simulink library "tqd"  (R2021b)
settings: Solver=VariableStepAuto  StartTime=0.0  StopTime=10.0  RelTol=1e-3
undefined symbols (not defined in the file): ATQD_AfterTqMinGain_X_Deg, ATQD_APSCreepBaseTqD_X_kph, ATQD_APSCreepBaseTqD_Y_Deg, ATQD_APSCreepBaseTqR_X_kph, ATQD_APSCreepBaseTqR_Y_Deg, ATQD_APSCreepIterm_X_kph, ATQD_APSCreepIterm_Y_kph, ATQD_APSCreepPterm_X_kph, ATQD_APSCreepPterm_Y_kph, ATQD_APSDecReq_X_kph, ATQD_APSDecReq_Y_mps2, ATQD_APSDecReqCMD_X_kph, ATQD_APSDecReqTs_X_pct, ATQD_APSDecTimeGain_X_Deg, ATQD_APSDecTimeGain_Y_s, ATQD_APSReqLowSpd_X_Deg, ATQD_AutoHoldReleaseBPS_X_Deg, ATQD_AWDLoadTrqnsGain_X_kg, ATQD_AWDLoadTrqnsGain_Y_pct, ATQD_BOSEnBPSPosn_X_kph, ATQD_BOSMap_X_rpm, ATQD_BOSMap_Y_pct, ATQD_CreepBaseTqD_X_kph, ATQD_CreepBaseTqD_Y_Deg, ATQD_CreepBaseTqR_X_kph, ATQD_CreepBaseTqR_Y_Deg, ATQD_CreepBPSDisPosn_X_Deg, ATQD_CreepBPSDisPosnR_X_Deg, ATQD_CreepBPSEnPosn_X_Deg, ATQD_CreepBPSEnPosnR_X_Deg, ATQD_CreepDeltaTq_X_kph, ATQD_CreepIterm_X_kph, ATQD_CreepIterm_Y_kph, ATQD_CreepItermMaxLimit_X_pct, ATQD_CreepPreloadTime_X_kph, ATQD_CreepPreloadTq_X_kph, ATQD_CreepPreloadTq_Y_s, ATQD_CreepProtTq_X_Deg, ATQD_CreepPterm_X_kph, ATQD_CreepPterm_Y_kph, ATQD_CreepRrTqSpRat_X_rpm, ATQD_CreepRrTqSpRat_Y_Nm, ATQD_CreepTargetSpdD_X_pct, ATQD_CreepTargetSpdR_X_pct, ATQD_ECOTqMapD_X_rpm, ATQD_ECOTqMapD_Y_pct, ATQD_EMTqMapD_X_rpm, ATQD_EMTqMapD_Y_pct, ATQD_EOPDTqMapDCon_X_rpm, ATQD_EOPDTqMapDCon_Y_Deg, ATQD_EscapeModePedTq_X_pct, ATQD_EscapeModePedTq_Y_rpm, ATQD_EscapeModePedTqFr_X_pct, ATQD_EscapeModePedTqFr_Y_rpm, ATQD_EstInitVehWeight_X_c, ATQD_FAfterTqCMDGain_X_rpm, ATQD_FAfterTqCMDGain_Y_pct, ATQD_FrLossMAPLowV_X_rpm, ATQD_FrLossMAPLowV_Y_Nm, ATQD_FrMotActReduce_X_rpm ... (+772)
libraries: simulink x211, hcu_lib x179, tqr x3
(part 19 of 28)

== system tqd/TQD/TorqueDemand/TorqueModule/AvaliableTqLimit/TorqueCapacityCalcalation/Generation ==
  VTQD_FrShaftSpd_rpm : Inport
  VTQD_RrShaftSpd_rpm : Inport  Port=2
  VTQD_FrHVBPwrAvailChrg_kw : Inport  Port=3
  VTQD_RrHVBPwrAvailChrg_kw : Inport  Port=4
  KTQD_FrBatapCont_factor : Inport  Port=5
  KTQD_RrBatapCont_factor : Inport  Port=6
  VINP_FrRegenAvailTq_Nm : Inport  Port=7
  VINP_RrRegenAvailTq_Nm : Inport  Port=8
  VTQD_GearActualPosn_enum : Inport  Port=9
  VINP_VehicleType_enum : Inport  Port=10
  VTQD_FrMotorTempHigh_flg : Inport  Port=11
  VTQD_RrMotorTempHigh_flg : Inport  Port=12
  VTQD_FrGenActReduce_Nm : Inport  Port=13
  VTQD_RrGenActReduce_Nm : Inport  Port=14
  Abs2 : Abs
  Abs6 : Abs
  Constant : Constant  Value=KTQD_WhlTqCapGenFr_Nm_ovrdflg
  Constant1 : Constant  Value=KTQD_WhlTqCapGenFr_Nm_ovrdval
  Constant10 : Constant  Value=ENUM_GEARACTUALPOSN_P  OutDataTypeStr=single
  Constant11 : Constant  Value=ENUM_VEHICLETYPE_D31L24
  Constant12 : Constant  Value=KTQD_RrLowTheldTrq_Nm  OutDataTypeStr=single
  Constant13 : Constant  Value=ZERO_FLOAT
  Constant14 : Constant  Value=KTQD_FrLowTheldTrq_Nm  OutDataTypeStr=single
  Constant15 : Constant  Value=KTQD_NewTotalCapTqSW_flg
  Constant16 : Constant  Value=ENUM_GEARACTUALPOSN_N  OutDataTypeStr=single
  Constant17 : Constant  Value=ENUM_GEARACTUALPOSN_P  OutDataTypeStr=single
  Constant18 : Constant  Value=KTQD_FrLowTheldTrq_Nm
  Constant19 : Constant  Value=ENUM_VEHICLETYPE_D31L24
  Constant2 : Constant  Value=KTQD_RrTMSpdMin_rpm  OutDataTypeStr=single
  Constant24 : Constant  Value=KTQD_NewTotalCapTqSW_flg
  Constant25 : Constant  Value=KTQD_RrLowTheldTrq_Nm
  Constant3 : Constant  Value=KTQD_WhlTqCapGenRr_Nm_ovrdflg
  Constant4 : Constant  Value=KTQD_RrTMTotalGearRatio_gain  OutDataTypeStr=single
  Constant5 : Constant  Value=KTQD_FrTMSpdMin_rpm  OutDataTypeStr=single
  Constant6 : Constant  Value=KTQD_FrTMTotalGearRatio_gain  OutDataTypeStr=single
  Constant7 : Constant  Value=KTQD_WhlTqCapGenRr_Nm_ovrdval
  Constant8 : Constant  Value=ZERO_FLOAT
  Constant9 : Constant  Value=ENUM_GEARACTUALPOSN_N  OutDataTypeStr=single
  Equal{1..4} (4 alike) : RelationalOperator  Operator===  OutDataTypeStr=boolean  RndMeth=Simplest
  Equal5 : RelationalOperator  Operator=~=  OutDataTypeStr=boolean  RndMeth=Simplest
  Equal6 : RelationalOperator  Operator=~=  OutDataTypeStr=boolean  RndMeth=Simplest
  Fcn : Fcn  Expr=u[1]/u[2]/pi*u[3]
  Fcn2 : Fcn  Expr=u[1]/u[2]/pi*u[3]
  Gain1 : Gain  Gain=-1
  Gain4 : Gain  Gain=-1
  Logical Operator1 : Logic  AllPortsSameDT=off  OutDataTypeStr=boolean
  Logical Operator2 : Logic  AllPortsSameDT=off  OutDataTypeStr=boolean
  Max{,1..5} (6 alike) : MinMax  Function=max  Inputs=2
  Mux : Mux  Inputs=3
  Mux2 : Mux  Inputs=3
  OR1 : Logic  Operator=OR  AllPortsSameDT=off  OutDataTypeStr=boolean
  OR2 : Logic  Operator=OR  AllPortsSameDT=off  OutDataTypeStr=boolean
  Product1 : Product
  Product2 : Product
  Saturation1 : Saturate  UpperLimit=0  LowerLimit=KTQD_FrLowTheldTrq_Nm
      settings: AttributesFormatString=|
      | Upper Limit :%<UpperLimit>
      | Lower Limit :%<LowerLimit>
  Saturation2 : Saturate  UpperLimit=0  LowerLimit=KTQD_RrLowTheldTrq_Nm
      settings: AttributesFormatString=|
      | Upper Limit :%<UpperLimit>
      | Lower Limit :%<LowerLimit>
  Switch{,1,6..7} (4 alike) : Switch  Criteria=u2 ~= 0
      Switch settings: AttributesFormatString=<%<Criteria>>
      Switch1 settings: AttributesFormatString=<%<Criteria>>
      Switch6 settings: AttributesFormatString=%<Criteria>
      Switch7 settings: AttributesFormatString=%<Criteria>
  Switch{2..5} (4 alike) : Switch  Criteria=u2 > Threshold
  VTQD_WhlTqCapGenFr_Nm : Outport
  VTQD_WhlTqCapGenRr_Nm : Outport  Port=2
  wires:
  Gain1/1 -> Saturation2/1
  Gain4/1 -> Saturation1/1
  Switch1/1 -> VTQD_WhlTqCapGenRr_Nm/1  "VTQD_WhlTqCapGenRr_Nm"
  Constant3/1 -> Switch1/2
  Constant7/1 -> Switch1/1
  Switch/1 -> VTQD_WhlTqCapGenFr_Nm/1  "VTQD_WhlTqCapGenFr_Nm"
  Constant1/1 -> Switch/1
  Constant/1 -> Switch/2
  VTQD_RrHVBPwrAvailChrg_kw/1 -> [VTQD_RrHVBPwrAvailChrg_kw]
  KTQD_FrBatapCont_factor/1 -> [KTQD_FrBatapCont_factor]
  VTQD_FrHVBPwrAvailChrg_kw/1 -> [VTQD_FrHVBPwrAvailChrg_kw]
  VTQD_FrShaftSpd_rpm/1 -> [VTQD_FrShaftSpd_rpm]
  VTQD_RrShaftSpd_rpm/1 -> [VTQD_RrShaftSpd_rpm]
  KTQD_RrBatapCont_factor/1 -> [KTQD_RrBatapCont_factor]
  Fcn2/1 -> Gain1/1
  Max1/1 -> Mux2/2
  Abs2/1 -> Max1/1
  Mux2/1 -> Fcn2/1
  Constant2/1 -> Max1/2
  [KTQD_RrBatapCont_factor] -> Mux2/3
  [VTQD_RrShaftSpd_rpm] -> Abs2/1
  [VTQD_RrHVBPwrAvailChrg_kw] -> Mux2/1
  Abs6/1 -> Max4/1
  [VTQD_FrHVBPwrAvailChrg_kw] -> Mux/1
  Constant5/1 -> Max4/2
  [VTQD_FrShaftSpd_rpm] -> Abs6/1
  [KTQD_FrBatapCont_factor] -> Mux/3
  Mux/1 -> Fcn/1
  Max4/1 -> Mux/2
  [VINP_FrRegenAvailTq_Nm] -> Product2/1
  Constant6/1 -> Product2/2
  [VINP_RrRegenAvailTq_Nm] -> Product1/1
  Constant4/1 -> Product1/2
  VINP_RrRegenAvailTq_Nm/1 -> [VINP_RrRegenAvailTq_Nm]
  VINP_FrRegenAvailTq_Nm/1 -> [VINP_FrRegenAvailTq_Nm]
  [VTQD_GearActualPosn_enum] -> Equal3/1
  Equal3/1 -> OR1/1
  Constant17/1 -> Equal3/2
  [VTQD_GearActualPosn_enum] -> Equal1/1
  Constant13/1 -> Switch3/1
  Equal1/1 -> OR1/2
  Constant16/1 -> Equal1/2
  Switch3/1 -> Max/2
  Constant8/1 -> Switch2/1
  [VTQD_GearActualPosn_enum] -> Equal2/1
  Constant10/1 -> Equal4/2
  Equal4/1 -> OR2/1
  Constant9/1 -> Equal2/2
  Equal2/1 -> OR2/2
  [VTQD_GearActualPosn_enum] -> Equal4/1
  Switch2/1 -> Max2/2
  VTQD_GearActualPosn_enum/1 -> [VTQD_GearActualPosn_enum]
  Max/1 -> Switch1/3
  Max2/1 -> Switch/3
  VINP_VehicleType_enum/1 -> [VINP_VehicleType_enum]
  Equal6/1 -> Logical Operator1/2
  [VINP_VehicleType_enum] -> Equal6/1
  Constant19/1 -> Equal6/2
  Logical Operator1/1 -> Switch2/2
  OR2/1 -> Logical Operator1/1
  [VINP_VehicleType_enum] -> Equal5/1
  Constant11/1 -> Equal5/2
  Equal5/1 -> Logical Operator2/2
  Logical Operator2/1 -> Switch3/2
  OR1/1 -> Logical Operator2/1
  VTQD_FrMotorTempHigh_flg/1 -> [VTQD_FrMotorTempHigh_flg]
  VTQD_RrMotorTempHigh_flg/1 -> [VTQD_RrMotorTempHigh_flg]
  VTQD_FrGenActReduce_Nm/1 -> [VTQD_FrGenActReduce_Nm]
  VTQD_RrGenActReduce_Nm/1 -> [VTQD_RrGenActReduce_Nm]
  [VTQD_RrGenActReduce_Nm] -> Switch4/1
  [VTQD_RrMotorTempHigh_flg] -> Switch4/2
  Product1/1 -> Max5/1
  Switch4/1 -> Max5/2
  Max5/1 -> Switch3/3
  [VTQD_FrMotorTempHigh_flg] -> Switch5/2
  [VTQD_FrGenActReduce_Nm] -> Switch5/1
  Max3/1 -> Switch2/3
  Product2/1 -> Max3/1
  Switch5/1 -> Max3/2
  Fcn/1 -> Gain4/1
  Constant14/1 -> Switch5/3
  Constant12/1 -> Switch4/3
  Constant25/1 -> Switch7/1
  Constant24/1 -> Switch7/2
  Saturation2/1 -> Switch7/3
  Switch7/1 -> Max/1
  Constant18/1 -> Switch6/1
  Constant15/1 -> Switch6/2
  Saturation1/1 -> Switch6/3
  Switch6/1 -> Max2/1

== system tqd/TQD/TorqueDemand/TorqueModule/AvaliableTqLimit/TorqueCapacityCalcalation/MOTOR Loss MAP  ==
  note: Determination
  note: Front Loss Power Calculation
  note: Calabration Parameters/Maps
  note: Rear Loss Power Calculation
  VTQD_FrShaftSpd_rpm : Inport
  VTQD_RrShaftSpd_rpm : Inport  Port=2
  VTQD_CoordWhlTqDemFr_Nm : Inport  Port=3
  VTQD_CoordWhlTqDemRr_Nm : Inport  Port=4
  VINP_FrMCUDCBusVolt_V : Inport  Port=5
  VINP_RrMCUDCBusVolt_V : Inport  Port=6
  VPMM_DrivetrainSelect_enum : Inport  Port=7
  AND : Logic  AllPortsSameDT=off  OutDataTypeStr=boolean
  AND2 : Logic  AllPortsSameDT=off  OutDataTypeStr=boolean
  Add : Sum
  Add2 : Sum
  Add3 : Sum
  Constant : Constant  Value=KTQD_FrLossMAPLowV_V
  Constant1 : Constant  Value=KTQD_FrLossMAPHighV_V
  Constant10 : Constant  Value=eps  OutDataTypeStr=single
  Constant{6,11..13} (4 alike) : Constant  Value=ZERO_FLOAT
  Constant2 : Constant  Value=KTQD_RrLossMAPLowV_V
  Constant3 : Constant  Value=KTQD_RrLossMAPHighV_V
  Constant4 : Constant  Value=ENUM_DRIVETRAIN_AWD
  Constant5 : Constant  Value=ENUM_DRIVETRAIN_RWD
  Constant7 : Constant  Value=eps  OutDataTypeStr=single
  Divide : Product  Inputs=*/
  Divide2 : Product  Inputs=*/
  Equal : RelationalOperator  Operator===  OutDataTypeStr=boolean  RndMeth=Simplest
  Equal1 : RelationalOperator  Operator===  OutDataTypeStr=boolean  RndMeth=Simplest
  GreaterThan : RelationalOperator  Operator=>  OutDataTypeStr=boolean  RndMeth=Simplest
  GreaterThan2 : RelationalOperator  Operator=>  OutDataTypeStr=boolean  RndMeth=Simplest
  Less Than : RelationalOperator  Operator=<  OutDataTypeStr=boolean  RndMeth=Simplest
  Less Than2 : RelationalOperator  Operator=<  OutDataTypeStr=boolean  RndMeth=Simplest
  MTQD_FrLossMAPHighV_Z_kw : Lookup_n-D  BreakpointsForDimension1=ATQD_FrLossMAPLowV_Y_Nm  BreakpointsForDimension2=ATQD_FrLossMAPLowV_X_rpm  Table=MTQD_FrLossMAPHighV_Z_kw  InternalRulePriority=Speed  RndMeth=Simplest  InputSameDT=on
      settings: InputPortMap=u0,u1
  MTQD_FrLossMAPLowV_Z_kw : Lookup_n-D  BreakpointsForDimension1=ATQD_FrLossMAPLowV_Y_Nm  BreakpointsForDimension2=ATQD_FrLossMAPLowV_X_rpm  Table=MTQD_FrLossMAPLowV_Z_kw  InternalRulePriority=Speed  RndMeth=Simplest  InputSameDT=on
      settings: InputPortMap=u0,u1
  MTQD_RrLossMAPHighV_Z_kw : Lookup_n-D  BreakpointsForDimension1=ATQD_RrLossMAPLowV_Y_Nm  BreakpointsForDimension2=ATQD_RrLossMAPLowV_X_rpm  Table=MTQD_RrLossMAPHighV_Z_kw  InternalRulePriority=Speed  RndMeth=Simplest  InputSameDT=on
      settings: InputPortMap=u0,u1
  MTQD_RrLossMAPLowV_Z_kw : Lookup_n-D  BreakpointsForDimension1=ATQD_RrLossMAPLowV_Y_Nm  BreakpointsForDimension2=ATQD_RrLossMAPLowV_X_rpm  Table=MTQD_RrLossMAPLowV_Z_kw  InternalRulePriority=Speed  RndMeth=Simplest  InputSameDT=on
      settings: InputPortMap=u0,u1
  Max : MinMax  Function=max  Inputs=2
  Max1 : MinMax  Function=max  Inputs=2
  Product : Product
  Product2 : Product
  Subtract{,1..2,6..8} (6 alike) : Sum  Inputs=+-
  Switch : Switch  Criteria=u2 > Threshold
  Switch1 : Switch  Criteria=u2 > Threshold
  Switch3 : Switch  Criteria=u2 ~= 0
  Switch4 : Switch  Criteria=u2 ~= 0
  VTQD_MotorLossTotal_kw : Outport
  wires:
  MTQD_FrLossMAPLowV_Z_kw/1 -> [VTQD_FrLossMAPLowV_kw]  "VTQD_FrLossMAPLowV_kw"
  MTQD_FrLossMAPHighV_Z_kw/1 -> [VTQD_FrLossMAPHighV_kw]  "VTQD_FrLossMAPHighV_kw"
  Constant/1 -> [VTQD_FrLossMAPLowV_V]  "VTQD_FrLossMAPLowV_V"
  Constant1/1 -> [VTQD_FrLossMAPHighV_V]  "VTQD_FrLossMAPHighV_V"
  Constant2/1 -> [VTQD_RrLossMAPLowV_V]  "VTQD_RrLossMAPLowV_V"
  Constant3/1 -> [VTQD_RrLossMAPHighV_V]  "VTQD_RrLossMAPHighV_V"
  MTQD_RrLossMAPLowV_Z_kw/1 -> [VTQD_RrLossMAPLowV_kw]  "VTQD_RrLossMAPLowV_kw"
  MTQD_RrLossMAPHighV_Z_kw/1 -> [VTQD_RrLossMAPHighV_kw]  "VTQD_RrLossMAPHighV_kw"
  VINP_FrMCUDCBusVolt_V/1 -> [VINP_FrMCUDCBusVolt_V]
  VINP_RrMCUDCBusVolt_V/1 -> [VINP_RrMCUDCBusVolt_V]
  [VINP_FrMCUDCBusVolt_V] -> Subtract/1
  [VTQD_FrLossMAPLowV_V] -> Subtract/2
  Subtract/1 -> Divide/1
  Divide/1 -> Product/1
  Product/1 -> Add/1
  [VTQD_FrLossMAPLowV_kw] -> Add/2
  Switch3/1 -> [VTQD_FrLossMAPFinal_kw]  "VTQD_FrLossMAPFinal_kw"
  [VPMM_DrivetrainSelect_enum] -> Equal/1
  Constant4/1 -> Equal/2
  Equal/1 -> Switch/2
  Add2/1 -> Switch/1
  [VPMM_DrivetrainSelect_enum] -> Equal1/1
  Constant5/1 -> Equal1/2
  [VTQD_RrLossMAPFinal_kw] -> Switch1/1
  Switch1/1 -> Switch/3
  [VTQD_FrLossMAPFinal_kw] -> Switch1/3
  Equal1/1 -> Switch1/2
  Switch/1 -> [VTQD_MotorLossTotal_kw]  "VTQD_MotorLossTotal_kw"
  VTQD_CoordWhlTqDemFr_Nm/1 -> [VTQD_CoordWhlTqDemFr_Nm]
  Add/1 -> Switch3/1
  [VTQD_CoordWhlTqDemFr_Nm] -> GreaterThan/1
  Constant6/1 -> GreaterThan/2
  GreaterThan/1 -> AND/1
  Constant11/1 -> Switch3/3
  Less Than/1 -> AND/2
  AND/1 -> Switch3/2
  VTQD_FrShaftSpd_rpm/1 -> [VTQD_FrShaftSpd_rpm]
  VTQD_RrShaftSpd_rpm/1 -> [VTQD_RrShaftSpd_rpm]
  VTQD_CoordWhlTqDemRr_Nm/1 -> [VTQD_CoordWhlTqDemRr_Nm]
  VPMM_DrivetrainSelect_enum/1 -> [VPMM_DrivetrainSelect_enum]
  [VTQD_CoordWhlTqDemFr_Nm] -> MTQD_FrLossMAPLowV_Z_kw/1
  [VTQD_FrShaftSpd_rpm] -> MTQD_FrLossMAPLowV_Z_kw/2
  [VTQD_CoordWhlTqDemFr_Nm] -> MTQD_FrLossMAPHighV_Z_kw/1
  [VTQD_FrShaftSpd_rpm] -> MTQD_FrLossMAPHighV_Z_kw/2
  [VTQD_CoordWhlTqDemRr_Nm] -> MTQD_RrLossMAPLowV_Z_kw/1
  [VTQD_RrShaftSpd_rpm] -> MTQD_RrLossMAPLowV_Z_kw/2
  [VTQD_CoordWhlTqDemRr_Nm] -> MTQD_RrLossMAPHighV_Z_kw/1
  [VTQD_RrShaftSpd_rpm] -> MTQD_RrLossMAPHighV_Z_kw/2
  [VTQD_FrLossMAPLowV_V] -> Subtract1/2
  [VTQD_FrLossMAPHighV_V] -> Subtract1/1
  Subtract1/1 -> Max/1
  Constant10/1 -> Max/2
  Max/1 -> Divide/2
  [VTQD_FrLossMAPLowV_kw] -> Subtract2/2
  [VTQD_FrLossMAPHighV_kw] -> Subtract2/1
  Subtract2/1 -> Product/2
  [VINP_FrMCUDCBusVolt_V] -> Less Than/1
  [VTQD_FrLossMAPHighV_V] -> Less Than/2
  [VTQD_RrLossMAPHighV_V] -> Less Than2/2
  [VINP_RrMCUDCBusVolt_V] -> Less Than2/1
  Subtract8/1 -> Product2/2
  [VTQD_RrLossMAPHighV_kw] -> Subtract8/1
  [VTQD_RrLossMAPLowV_kw] -> Subtract8/2
  Max1/1 -> Divide2/2
  Constant7/1 -> Max1/2
  Subtract7/1 -> Max1/1
  [VTQD_RrLossMAPHighV_V] -> Subtract7/1
  [VTQD_RrLossMAPLowV_V] -> Subtract7/2
  AND2/1 -> Switch4/2
  Less Than2/1 -> AND2/2
  Constant12/1 -> Switch4/3
  GreaterThan2/1 -> AND2/1
  Constant13/1 -> GreaterThan2/2
  [VTQD_CoordWhlTqDemRr_Nm] -> GreaterThan2/1
  Add3/1 -> Switch4/1
  Switch4/1 -> [VTQD_RrLossMAPFinal_kw]  "VTQD_RrLossMAPFinal_kw"
  [VTQD_RrLossMAPLowV_kw] -> Add3/2
  Product2/1 -> Add3/1
  Divide2/1 -> Product2/1
  Subtract6/1 -> Divide2/1
  [VTQD_RrLossMAPLowV_V] -> Subtract6/2
  [VINP_RrMCUDCBusVolt_V] -> Subtract6/1
  [VTQD_FrLossMAPFinal_kw] -> Add2/1
  [VTQD_RrLossMAPFinal_kw] -> Add2/2
  [VTQD_MotorLossTotal_kw] -> VTQD_MotorLossTotal_kw/1

== system tqd/TQD/TorqueDemand/TorqueModule/AvaliableTqLimit/TorqueCapacityCalcalation/Motoring ==
  VTQD_FrShaftSpd_rpm : Inport
  VTQD_RrShaftSpd_rpm : Inport  Port=2
  VTQD_FrHVBPwrAvailDchrg_kw : Inport  Port=3
  VTQD_RrHVBPwrAvailDchrg_kw : Inport  Port=4
  KTQD_FrBatapCont_factor : Inport  Port=5
  KTQD_RrBatapCont_factor : Inport  Port=6
  VINP_FrMotorAvailTq_Nm : Inport  Port=7
  VINP_RrMotorAvailTq_Nm : Inport  Port=8
  VTQD_GearActualPosn_enum : Inport  Port=9
  VINP_VehicleType_enum : Inport  Port=10
  VTQD_FrMotorTempHigh_flg : Inport  Port=11
  VTQD_RrMotorTempHigh_flg : Inport  Port=12
  VTQD_FrMotActReduce_gain : Inport  Port=13
  VTQD_RrMotActReduce_Nm : Inport  Port=14
  VTQD_FrRockDisAvalMotTq_Nm : Inport  Port=15
  VTQD_RrRockDisAvalMotTq_Nm : Inport  Port=16
  Abs : Abs
  Abs2 : Abs
  Constant : Constant  Value=KTQD_WhlTqCapMotFr_Nm_ovrdflg
  Constant1 : Constant  Value=KTQD_FrTMSpdMin_rpm  OutDataTypeStr=single
  Constant10 : Constant  Value=KTQD_FrTMTotalGearRatio_gain  OutDataTypeStr=single
  Constant11 : Constant  Value=KTQD_RrTMTotalGearRatio_gain  OutDataTypeStr=single
  Constant{2,4,12..13} (4 alike) : Constant  Value=ZERO_FLOAT
  Constant14 : Constant  Value=ENUM_GEARACTUALPOSN_N  OutDataTypeStr=single
  Constant15 : Constant  Value=ENUM_GEARACTUALPOSN_P  OutDataTypeStr=single
  Constant16 : Constant  Value=ENUM_GEARACTUALPOSN_N  OutDataTypeStr=single
  Constant17 : Constant  Value=ENUM_GEARACTUALPOSN_P  OutDataTypeStr=single
  Constant18 : Constant  Value=ENUM_VEHICLETYPE_D31L24
  Constant19 : Constant  Value=ENUM_VEHICLETYPE_D31L24
  Constant20 : Constant  Value=KTQD_RrUppTheldTrq_Nm
  Constant21 : Constant  Value=KTQD_FrUppTheldTrq_Nm
  Constant22 : Constant  Value=KTQD_NewTotalCapTqSW_flg
  Constant23 : Constant  Value=KTQD_FrUppTheldTrq_Nm
  Constant24 : Constant  Value=KTQD_NewTotalCapTqSW_flg
  Constant25 : Constant  Value=KTQD_RrUppTheldTrq_Nm
  Constant3 : Constant  Value=KTQD_RrTMSpdMin_rpm  OutDataTypeStr=single
  Constant5 : Constant  Value=KTQD_WhlTqCapMotFr_Nm_ovrdval
  Constant6 : Constant  Value=KTQD_WhlTqCapMotRr_Nm_ovrdflg
  Constant7 : Constant  Value=KTQD_WhlTqCapMotRr_Nm_ovrdval
  Constant8 : Constant  Value=KTQD_FrUppTheldTrq_Nm
  Constant9 : Constant  Value=KTQD_RrUppTheldTrq_Nm
  Equal{,1..3} (4 alike) : RelationalOperator  Operator===  OutDataTypeStr=boolean  RndMeth=Simplest
  Equal4 : RelationalOperator  Operator=~=  OutDataTypeStr=boolean  RndMeth=Simplest
  Equal6 : RelationalOperator  Operator=~=  OutDataTypeStr=boolean  RndMeth=Simplest
  Fcn : Fcn  Expr=u[1]/u[2]/pi*u[3]
  Fcn2 : Fcn  Expr=u[1]/u[2]/pi*u[3]
  Logical Operator1 : Logic  AllPortsSameDT=off  OutDataTypeStr=boolean
  Logical Operator2 : Logic  AllPortsSameDT=off  OutDataTypeStr=boolean
  Max{,1..3} (4 alike) : MinMax  Function=max  Inputs=2
  Min : MinMax  Inputs=4
  Min1 : MinMax  Inputs=4
  Min2 : MinMax  Inputs=2
  Min3 : MinMax  Inputs=2
  Mux : Mux  Inputs=3
  Mux2 : Mux  Inputs=3
  OR : Logic  Operator=OR  AllPortsSameDT=off  OutDataTypeStr=boolean
  OR1 : Logic  Operator=OR  AllPortsSameDT=off  OutDataTypeStr=boolean
  Product : Product
  Product1 : Product
  Switch{,1,6..7} (4 alike) : Switch  Criteria=u2 ~= 0
      Switch settings: AttributesFormatString=<%<Criteria>>
      Switch1 settings: AttributesFormatString=<%<Criteria>>
      Switch6 settings: AttributesFormatString=%<Criteria>
      Switch7 settings: AttributesFormatString=%<Criteria>
  Switch{2..5} (4 alike) : Switch  Criteria=u2 > Threshold
  VTQD_WhlTqCapMotFr_Nm : Outport
  VTQD_WhlTqCapMotRr_Nm : Outport  Port=2
  wires:
  Switch1/1 -> VTQD_WhlTqCapMotRr_Nm/1  "VTQD_WhlTqCapMotRr_Nm"
  Constant7/1 -> Switch1/1
  Constant6/1 -> Switch1/2
  Constant5/1 -> Switch/1
  Constant/1 -> Switch/2
  Switch/1 -> VTQD_WhlTqCapMotFr_Nm/1  "VTQD_WhlTqCapMotFr_Nm"
  VTQD_RrHVBPwrAvailDchrg_kw/1 -> [VTQD_RrHVBPwrAvailDchrg_kw]
  KTQD_RrBatapCont_factor/1 -> [KTQD_RrBatapCont_factor]
  VTQD_RrShaftSpd_rpm/1 -> [VTQD_RrShaftSpd_rpm]
  Abs2/1 -> Max2/1
  [VTQD_RrHVBPwrAvailDchrg_kw] -> Mux2/1
  Constant3/1 -> Max2/2
  [VTQD_RrShaftSpd_rpm] -> Abs2/1
  Mux2/1 -> Fcn2/1
  Max2/1 -> Mux2/2
  [VTQD_FrHVBPwrAvailDchrg_kw] -> Mux/1
  Max/1 -> Mux/2
  [VTQD_FrShaftSpd_rpm] -> Abs/1
  KTQD_FrBatapCont_factor/1 -> [KTQD_FrBatapCont_factor]
  VTQD_FrHVBPwrAvailDchrg_kw/1 -> [VTQD_FrHVBPwrAvailDchrg_kw]
  Abs/1 -> Max/1
  Mux/1 -> Fcn/1
  VTQD_FrShaftSpd_rpm/1 -> [VTQD_FrShaftSpd_rpm]
  Constant1/1 -> Max/2
  Constant8/1 -> Min/2
  Min/1 -> Max1/1
  Constant2/1 -> Max1/2
  Constant9/1 -> Min1/2
  Constant4/1 -> Max3/2
  [KTQD_FrBatapCont_factor] -> Mux/3
  [KTQD_RrBatapCont_factor] -> Mux2/3
  VINP_FrMotorAvailTq_Nm/1 -> [VINP_FrMotorAvailTq_Nm]
  VINP_RrMotorAvailTq_Nm/1 -> [VINP_RrMotorAvailTq_Nm]
  Constant10/1 -> Product/2
  [VINP_FrMotorAvailTq_Nm] -> Product/1
  [VINP_RrMotorAvailTq_Nm] -> Product1/1
  Constant11/1 -> Product1/2
  Min1/1 -> Max3/1
  Constant12/1 -> Switch2/1
  Constant14/1 -> Equal/2
  [VTQD_GearActualPosn_enum] -> Equal/1
  Equal2/1 -> OR/1
  [VTQD_GearActualPosn_enum] -> Equal2/1
  Equal/1 -> OR/2
  Constant15/1 -> Equal2/2
  Equal1/1 -> OR1/2
  Equal3/1 -> OR1/1
  Constant17/1 -> Equal3/2
  [VTQD_GearActualPosn_enum] -> Equal1/1
  Constant16/1 -> Equal1/2
  Constant13/1 -> Switch3/1
  [VTQD_GearActualPosn_enum] -> Equal3/1
  VTQD_GearActualPosn_enum/1 -> [VTQD_GearActualPosn_enum]
  Max1/1 -> Switch/3
  Max3/1 -> Switch1/3
  Constant19/1 -> Equal6/2
  [VINP_VehicleType_enum] -> Equal6/1
  Equal6/1 -> Logical Operator1/2
  VINP_VehicleType_enum/1 -> [VINP_VehicleType_enum]
  Logical Operator1/1 -> Switch2/2
  OR/1 -> Logical Operator1/1
  Equal4/1 -> Logical Operator2/2
  [VINP_VehicleType_enum] -> Equal4/1
  Constant18/1 -> Equal4/2
  Logical Operator2/1 -> Switch3/2
  OR1/1 -> Logical Operator2/1
  VTQD_RrMotActReduce_Nm/1 -> [VTQD_RrMotActReduce_Nm]
  VTQD_FrMotActReduce_gain/1 -> [VTQD_FrMotActReduce_Nm]
  VTQD_RrMotorTempHigh_flg/1 -> [VTQD_RrMotorTempHigh_flg]
  VTQD_FrMotorTempHigh_flg/1 -> [VTQD_FrMotorTempHigh_flg]
  [VTQD_RrMotorTempHigh_flg] -> Switch4/2
  [VTQD_RrMotActReduce_Nm] -> Switch4/1
  Product1/1 -> Min3/1
  Switch4/1 -> Min3/2
  Min3/1 -> Switch3/3
  [VTQD_FrMotorTempHigh_flg] -> Switch5/2
  [VTQD_FrMotActReduce_Nm] -> Switch5/1
  Product/1 -> Min2/1
  Switch5/1 -> Min2/2
  Min2/1 -> Switch2/3
  Constant21/1 -> Switch5/3
  Constant20/1 -> Switch4/3
  VTQD_FrRockDisAvalMotTq_Nm/1 -> [VTQD_FrRockDisAvalMotTq_Nm]
  VTQD_RrRockDisAvalMotTq_Nm/1 -> [VTQD_RrRockDisAvalMotTq_Nm]
  Switch2/1 -> Min/4
  [VTQD_FrRockDisAvalMotTq_Nm] -> Min/3
  Switch3/1 -> Min1/4
  [VTQD_RrRockDisAvalMotTq_Nm] -> Min1/3
  Fcn/1 -> Switch6/3
  Switch6/1 -> Min/1
  Constant23/1 -> Switch6/1
  Constant22/1 -> Switch6/2
  Constant24/1 -> Switch7/2
  Constant25/1 -> Switch7/1
  Fcn2/1 -> Switch7/3
  Switch7/1 -> Min1/1

== system tqd/TQD/TorqueDemand/TorqueModule/AvaliableTqLimit/TorqueCapacityCalcalation/TMAvailablePwr_Calculation ==
  VINP_HVBPwrAvailDchrg_kw : Inport
  Add : Sum
  Constant : Constant  Value=KTQD_DCDCCalPwrAvailRsv_kW
  Constant1 : Constant  Value=KTQD_THCMCalPwrAvailRsv_kW
  Constant2 : Constant  Value=KTQD_TMPwrAvailDchrg_kW_ovrdflg
  Constant3 : Constant  Value=ZERO_FLOAT
  Min : MinMax  Function=max  Inputs=2
  Subtract : Sum  Inputs=+-
  Switch : Switch  Criteria=u2 ~= 0
      settings: AttributesFormatString=<%<Criteria>>
  VTQD_TMPwrAvailDchrg_kW : Outport
  wires:
  Constant3/1 -> Min/2
  Min/1 -> Switch/1
  Switch/1 -> VTQD_TMPwrAvailDchrg_kW/1  "VTQD_TMPwrAvailDchrg_kW"
  Constant2/1 -> Switch/2
  Subtract/1 -> Min/1
  Add/1 -> Subtract/2
  VINP_HVBPwrAvailDchrg_kw/1 -> Subtract/1, Switch/3
  Constant1/1 -> Add/2
  Constant/1 -> Add/1

== system tqd/TQD/TorqueDemand/TorqueModule/DriverWhlTqDem/Creep/If Action Subsystem ==
  In1 : Inport
  Action Port : ActionPort
  Out1 : Outport
  wires:
  In1/1 -> Out1/1

== system tqd/TQD/TorqueDemand/TorqueModule/DriverWhlTqDem/Creep/If Action Subsystem1 ==
  VTQD_ActBPSPosnInRange_flg : Inport
  VTQD_CreepPtermInp_c : Inport  Port=2
  VTQD_CreepItermInp_c : Inport  Port=3
  VTQD_CreepDeltaTq_Nm : Inport  Port=4
  VTQD_ActBPSPosn_pct : Inport  Port=5
  VTQD_CreepDisable_flg : Inport  Port=6
  VTQD_CreepEnable_flg : Inport  Port=7
  VTQD_OPDOn2Off_flg : Inport  Port=8
  VTQD_LowSkipDisCreep_flg : Inport  Port=9
  VVMC_APSActive_flg : Inport  Port=10
  Add : Sum
  Add1 : Sum  Inputs=+++
  Constant : Constant  Value=ZERO_FLOAT
  Constant1 : Constant  Value=KTQD_CreepItermMinLimit_Nm
  Constant2 : Constant  Value=KTQD_APSCreepItermMaxLim_Nm
  Constant4 : Constant  Value=ZERO_FLOAT
  Constant5 : Constant  Value=ONE_FLOAT
  Constant87 : Constant  Value=KTQD_APSCreepParOvrd_flg
  Data Type Conversion : DataTypeConversion
  MTQD_CreepItermMaxLimit_Y_Nm : Lookup_n-D  NumberOfTableDimensions=1  BreakpointsForDimension1=ATQD_CreepItermMaxLimit_X_pct  Table=MTQD_CreepItermMaxLimit_Y_Nm  ExtrapMethod=Clip  InternalRulePriority=Speed  RndMeth=Simplest  InputSameDT=on
  NOT : Logic  Operator=NOT  AllPortsSameDT=off  OutDataTypeStr=boolean
  OR : Logic  Operator=OR  Inputs=5  AllPortsSameDT=off  OutDataTypeStr=boolean
  OR19 : Logic  Operator=OR  AllPortsSameDT=off  OutDataTypeStr=boolean
  Product : Product
  Product2 : Product
  Saturation Dynamic : simulink/Discontinuities/Saturation Dynamic  OutMin=[]  OutMax=[]  OutDataTypeStr=Inherit: Same as second input  OutDataType=fixdt(1, 16)  OutScaling=2^-10  DoSatur=off
  Switch : Switch  Criteria=u2 ~= 0
      settings: AttributesFormatString=%<Criteria>
  Switch1 : Switch  Criteria=u2 ~= 0
  Switch4 : Switch  Criteria=u2 ~= 0
  Unit Delay : UnitDelay  SampleTime=-1  HasFrameUpgradeWarning=on
  VTQD_CreepTotalOfstTq_Nm : Outport
  wires:
  Add1/1 -> VTQD_CreepTotalOfstTq_Nm/1  "VTQD_CreepTotalOfstTq_Nm"
  VTQD_CreepDeltaTq_Nm/1 -> [VTQD_CreepDeltaTq_Nm]
  VTQD_CreepItermInp_c/1 -> [VTQD_CreepItermInp_c]
  VTQD_CreepPtermInp_c/1 -> [VTQD_CreepPtermInp_c]
  VTQD_ActBPSPosnInRange_flg/1 -> [VTQD_ActBPSPosnInRange_flg]
  VTQD_ActBPSPosn_pct/1 -> [VTQD_ActBPSPosn_pct]
  VTQD_CreepDisable_flg/1 -> [VTQD_CreepDisable_flg]
  OR/1 -> [VTQD_CreepPICtrlReset_flg]  "VTQD_CreepPICtrlReset_flg"
  VTQD_CreepEnable_flg/1 -> [VTQD_CreepEnable_flg]
  [VTQD_OPDOn2Off_flg] -> OR/2
  [VTQD_CreepDisable_flg] -> OR/3
  [VTQD_ActBPSPosnInRange_flg] -> OR/1
  [VTQD_CreepEnable_flg] -> NOT/1
  NOT/1 -> OR/4
  Data Type Conversion/1 -> Add1/3  "VTQD_CreepOffsetTq_Nm"
  Constant1/1 -> Saturation Dynamic/3
  [VTQD_ActBPSPosn_pct] -> MTQD_CreepItermMaxLimit_Y_Nm/1
  [VTQD_CreepPICtrlReset_flg] -> Switch4/2
  Constant/1 -> Switch1/1
  Product/1 -> Switch1/3
  [VTQD_CreepPtermInp_c] -> Product/1
  Constant5/1 -> Product/2, Product2/1
  [VTQD_CreepPICtrlReset_flg] -> Switch1/2
  Add/1 -> Switch4/3
  Switch1/1 -> Add1/1  "VTQD_CreepPtermTq_Nm"
  Saturation Dynamic/1 -> Add1/2  "VTQD_CreepItermTq_Nm"
  Product2/1 -> Add/1
  Switch4/1 -> Unit Delay/1, Saturation Dynamic/2
  Unit Delay/1 -> Add/2
  Constant4/1 -> Switch4/1
  [VTQD_CreepItermInp_c] -> Product2/2
  [VTQD_CreepDeltaTq_Nm] -> Data Type Conversion/1
  VTQD_OPDOn2Off_flg/1 -> [VTQD_OPDOn2Off_flg]
  VTQD_LowSkipDisCreep_flg/1 -> [VTQD_LowSkipDisCreep_flg]
  [VTQD_LowSkipDisCreep_flg] -> OR/5
  VVMC_APSActive_flg/1 -> [VVMC_APSActive_flg]
  MTQD_CreepItermMaxLimit_Y_Nm/1 -> Switch/3
  Switch/1 -> Saturation Dynamic/1  "VTQD_CreepItermMaxLimit_Nm"
  Constant87/1 -> OR19/2
  [VVMC_APSActive_flg] -> OR19/1
  OR19/1 -> Switch/2
  Constant2/1 -> Switch/1

== system tqd/TQD/TorqueDemand/TorqueModule/DriverWhlTqDem/Creep/Switch Case Action Subsystem ==
  In1 : Inport
  Action Port : ActionPort
  Out1 : Outport
  wires:
  In1/1 -> Out1/1

== system tqd/TQD/TorqueDemand/TorqueModule/DriverWhlTqDem/DriverTqCoordination/New Preload Torque ==
  VTQD_PreLoadHold_flg : Inport
  VTQD_PreLoadHoldtime_s : Inport  Port=2
  VTQD_FrShaftSpd_rpm : Inport  Port=3
  VTQD_RrShaftSpd_rpm : Inport  Port=4
  AND1 : Logic  AllPortsSameDT=off  OutDataTypeStr=boolean
  AND3 : Logic  AllPortsSameDT=off  OutDataTypeStr=boolean
  Abs1 : Abs
  Abs2 : Abs
  Constant1 : Constant  Value=KTQD_PreLoadTqHold_rpm
  Constant16 : Constant  Value=KTQD_PreLoadTqHold_rpm
  Constant17 : Constant  Value=ZERO_FLOAT
  Constant2 : Constant  Value=ZERO_FLOAT
  MTQD_FrPreLoadTq_Y_Nm : Lookup_n-D  NumberOfTableDimensions=1  BreakpointsForDimension1=ATQD_FrPreLoadTq_X_s  Table=MTQD_FrPreLoadTq_Y_Nm  ExtrapMethod=Clip  InternalRulePriority=Speed  RndMeth=Simplest  InputSameDT=on
  MTQD_RrPreLoadTq_Y_Nm : Lookup_n-D  NumberOfTableDimensions=1  BreakpointsForDimension1=ATQD_FrPreLoadTq_X_s  Table=MTQD_RrPreLoadTq_Y_Nm  ExtrapMethod=Clip  InternalRulePriority=Speed  RndMeth=Simplest  InputSameDT=on
  NOT1 : Logic  Operator=NOT  AllPortsSameDT=off  OutDataTypeStr=boolean
  NOT6 : Logic  Operator=NOT  AllPortsSameDT=off  OutDataTypeStr=boolean
  Relational Operator1 : RelationalOperator  Operator=>  OutDataTypeStr=boolean  RndMeth=Simplest
  Relational Operator4 : RelationalOperator  Operator=>  OutDataTypeStr=boolean  RndMeth=Simplest
  SR_Latch1 : hcu_lib/Basic_Blocks/SR_Latch
  SR_Latch4 : hcu_lib/Basic_Blocks/SR_Latch
  Switch1 : Switch  Criteria=u2 ~= 0
  Switch6 : Switch  Criteria=u2 ~= 0
  VTQD_FrPreloadTq_Nm : Outport
  VTQD_RrPreloadTq_Nm : Outport  Port=2
  wires:
  [VTQD_FrShaftSpd_rpm] -> Abs2/1
  Switch6/1 -> [VTQD_FrPreloadTq_Nm]  "VTQD_FrPreloadTq_Nm"
  Constant17/1 -> Switch6/1
  Abs2/1 -> Relational Operator4/1
  Relational Operator4/1 -> AND3/2
  AND3/1 -> SR_Latch4/1
  NOT6/1 -> SR_Latch4/2
  [VTQD_PreLoadHoldtime_s] -> MTQD_FrPreLoadTq_Y_Nm/1
  MTQD_FrPreLoadTq_Y_Nm/1 -> Switch6/3
  SR_Latch4/1 -> Switch6/2
  [VTQD_PreLoadHold_flg] -> NOT6/1
  Constant16/1 -> Relational Operator4/2
  [VTQD_PreLoadHold_flg] -> AND3/1
  [VTQD_PreLoadHold_flg] -> NOT1/1
  [VTQD_PreLoadHold_flg] -> AND1/1
  Constant1/1 -> Relational Operator1/2
  AND1/1 -> SR_Latch1/1
  Relational Operator1/1 -> AND1/2
  Abs1/1 -> Relational Operator1/1
  NOT1/1 -> SR_Latch1/2
  [VTQD_PreLoadHoldtime_s] -> MTQD_RrPreLoadTq_Y_Nm/1
  Constant2/1 -> Switch1/1
  MTQD_RrPreLoadTq_Y_Nm/1 -> Switch1/3
  Switch1/1 -> [VTQD_RrPreloadTq_Nm]  "VTQD_RrPreloadTq_Nm"
  [VTQD_RrShaftSpd_rpm] -> Abs1/1
  SR_Latch1/1 -> Switch1/2
  VTQD_PreLoadHold_flg/1 -> [VTQD_PreLoadHold_flg]
  VTQD_PreLoadHoldtime_s/1 -> [VTQD_PreLoadHoldtime_s]
  VTQD_FrShaftSpd_rpm/1 -> [VTQD_FrShaftSpd_rpm]
  VTQD_RrShaftSpd_rpm/1 -> [VTQD_RrShaftSpd_rpm]
  [VTQD_FrPreloadTq_Nm] -> VTQD_FrPreloadTq_Nm/1
  [VTQD_RrPreloadTq_Nm] -> VTQD_RrPreloadTq_Nm/1

== system tqd/TQD/TorqueDemand/TorqueModule/DriverWhlTqDem/PedalMapWhlTq/LHM ==
  VTQD_ActAPSPosn_pct : Inport
  VTQD_TqTargetShaftSpd_rpm : Inport  Port=2
  VTQD_GearActualPosn_enum : Inport  Port=3
  VDDM_VehMalfunLevel_enum : Inport  Port=4
  VVMC_EstSlope_Deg : Inport  Port=5
  VTQD_VehActSpd_kph : Inport  Port=6
  Action Port : ActionPort
  Constant : Constant  Value=ZERO_FLOAT
  Constant1 : Constant  Value=ENUM_GEARACTUALPOSN_D
  Constant2 : Constant  Value=ENUM_GEARACTUALPOSN_R
  Constant3 : Constant  Value=ENUM_VEHMALFUNLEVEL_LEVEL2
  Constant5 : Constant  Value=ZERO_FLOAT
  Constant6 : Constant  Value=ZERO_FLOAT
  Equal1 : RelationalOperator  Operator===  OutDataTypeStr=boolean  RndMeth=Simplest
  Equal2 : RelationalOperator  Operator===  OutDataTypeStr=boolean  RndMeth=Simplest
  MTQD_LHMGrade2TqUpLim_Z_Nm : Lookup_n-D  BreakpointsForDimension1=ATQD_LHMGrade2TqUpLim_Y_Deg  BreakpointsForDimension2=ATQD_LHMGrade2TqUpLim_X_kph  Table=MTQD_LHMGrade2TqUpLim_Z_Nm  ExtrapMethod=Clip  InternalRulePriority=Speed  RndMeth=Simplest  InputSameDT=on
      settings: InputPortMap=u0,u1
  MTQD_NL1TqMapD_Z_Nm : Lookup_n-D  BreakpointsForDimension1=ATQD_NL1TqMapD_Y_pct  BreakpointsForDimension2=ATQD_NL1TqMapD_X_rpm  Table=MTQD_NL1TqMapD_Z_Nm  ExtrapMethod=Clip  InternalRulePriority=Speed  RndMeth=Simplest  InputSameDT=on
      settings: InputPortMap=u0,u1
  MTQD_NRMTqMapR_Z_Nm : Lookup_n-D  BreakpointsForDimension1=ATQD_NL1TqMapD_Y_pct  BreakpointsForDimension2=ATQD_NL1TqMapD_X_rpm  Table=MTQD_NRMTqMapR_Z_Nm  ExtrapMethod=Clip  InternalRulePriority=Speed  RndMeth=Simplest  InputSameDT=on
      settings: InputPortMap=u0,u1
  Relational Operator : RelationalOperator  Operator=>  OutDataTypeStr=boolean  RndMeth=Simplest
  Saturation Dynamic : simulink/Discontinuities/Saturation Dynamic  OutMin=[]  OutMax=[]  OutDataTypeStr=Inherit: Same as second input  OutDataType=fixdt(1, 16)  OutScaling=2^-10  DoSatur=off
  Switch1 : Switch  Criteria=u2 ~= 0
  Switch2 : Switch  Criteria=u2 ~= 0
  Switch4 : Switch  Criteria=u2 ~= 0
  VTQD_PedalMapWhlTqLHM_Nm : Outport
  wires:
  Switch4/1 -> VTQD_PedalMapWhlTqLHM_Nm/1
  Constant/1 -> Switch2/3
  [VTQD_LHMTqMapR_Nm] -> Switch2/1
  Equal2/1 -> Switch2/2
  Constant2/1 -> Equal2/2
  [VTQD_GearActualPosn_enum] -> Equal2/1
  Switch2/1 -> Switch1/3
  [VTQD_LHMTqMapD_Nm] -> Switch1/1
  Constant1/1 -> Equal1/2
  Equal1/1 -> Switch1/2
  [VTQD_GearActualPosn_enum] -> Equal1/1
  VTQD_GearActualPosn_enum/1 -> [VTQD_GearActualPosn_enum]
  VTQD_TqTargetShaftSpd_rpm/1 -> [VTQD_TqTargetShaftSpd_rpm]
  VTQD_ActAPSPosn_pct/1 -> [VTQD_ActAPSPosn_pct]
  VDDM_VehMalfunLevel_enum/1 -> [VDDM_VehMalfunLevel_enum]
  VVMC_EstSlope_Deg/1 -> [VVMC_EstSlope_Deg]
  VTQD_VehActSpd_kph/1 -> [VTQD_VehActSpd_kph]
  [VDDM_VehMalfunLevel_enum] -> Relational Operator/1
  MTQD_NRMTqMapR_Z_Nm/1 -> [VTQD_LHMTqMapR_Nm]  "VTQD_LHMTqMapR_Nm"
  [VTQD_TqTargetShaftSpd_rpm] -> MTQD_NL1TqMapD_Z_Nm/2
  [VVMC_EstSlope_Deg] -> MTQD_LHMGrade2TqUpLim_Z_Nm/1
  Constant3/1 -> Relational Operator/2
  MTQD_LHMGrade2TqUpLim_Z_Nm/1 -> [VTQD_LHMGrade2TqUpLim_Nm]  "VTQD_LHMGrade2TqUpLim_Nm"
  [VTQD_ActAPSPosn_pct] -> MTQD_NL1TqMapD_Z_Nm/1
  [VTQD_VehActSpd_kph] -> MTQD_LHMGrade2TqUpLim_Z_Nm/2
  [VTQD_TqTargetShaftSpd_rpm] -> MTQD_NRMTqMapR_Z_Nm/2
  [VTQD_ActAPSPosn_pct] -> MTQD_NRMTqMapR_Z_Nm/1
  Relational Operator/1 -> [VTQD_LHMPedTqForce0_flg]  "VTQD_LHMPedTqForce0_flg"
  MTQD_NL1TqMapD_Z_Nm/1 -> [VTQD_LHMTqMapD_Nm]  "VTQD_LHMTqMapD_Nm"
  [VTQD_LHMPedTqForce0_flg] -> Switch4/2
  Constant6/1 -> Switch4/1
  Switch1/1 -> Saturation Dynamic/2
  Saturation Dynamic/1 -> Switch4/3
  [VTQD_LHMGrade2TqUpLim_Nm] -> Saturation Dynamic/1
  Constant5/1 -> Saturation Dynamic/3

== system tqd/TQD/TorqueDemand/TorqueModule/DriverWhlTqDem/PedalMapWhlTq/NoLHM ==
  VTQD_ActAPSPosn_pct : Inport
  VTQD_TqTargetShaftSpd_rpm : Inport  Port=2
  VTQD_RegenMode_enum : Inport  Port=3
  VTQD_RollRegenEnable_flg : Inport  Port=4
  VTQD_RollingShaftSpd_rpm : Inport  Port=5
  VTQD_GearActualPosn_enum : Inport  Port=6
  VTQD_EVDriveMode_enum : Inport  Port=7
  VVMC_EstSlope_Deg : Inport  Port=8
  VTQD_APSReqTimer_s : Inport  Port=9
  VTQD_LowIdleAccPedal_flg : Inport  Port=10
  VTQD_OPDHoldEnRel_flg : Inport  Port=11
  VTQD_OPDHoldActRelTq_Nm : Inport  Port=12
  VTQD_VehActSpd_kph : Inport  Port=13
  VTQD_SlopeUp_flg : Inport  Port=14
  VINP_IVISnowModeCmd_flg : Inport  Port=15
  VTQD_IVIRockModeEn_flg : Inport  Port=16
  VTQD_PreDecTqLowLim_Nm : Inport  Port=17
  VTQD_BrkSwSta_flg : Inport  Port=18
  VTQD_CreepEnable_flg : Inport  Port=19
  Action Port : ActionPort  ActionPortLabel=else
  Constant11 : Constant  Value=ENUM_GEARACTUALPOSN_D
  Constant12 : Constant  Value=ENUM_GEARACTUALPOSN_R
  Equal7 : RelationalOperator  Operator===  OutDataTypeStr=boolean  RndMeth=Simplest
  Equal8 : RelationalOperator  Operator===  OutDataTypeStr=boolean  RndMeth=Simplest
  GearShiftCheck : If  NumInputs=2  IfExpression=u1~= 0  ElseIfExpressions=u2~= 0
  Merge1 : Merge  Inputs=3
  ShiftD : Subsystem  TreatAsAtomicUnit=on
  ShiftPorN : Subsystem  TreatAsAtomicUnit=on
  ShiftR : Subsystem  TreatAsAtomicUnit=on
  VTQD_PedalMapWhlTqNoLHM_Nm : Outport
  wires:
  [VTQD_RollingShaftSpd_rpm] -> ShiftD/6(VTQD_RollingShaftSpd_rpm)
  [VTQD_RollRegenEnable_flg] -> ShiftD/5(VTQD_RollRegenEnable_flg)
  ShiftR/1(VTQD_PedalMapWhlTqR_Nm) -> Merge1/2
  VTQD_EVDriveMode_enum/1 -> [VTQD_EVDriveMode_enum]
  VTQD_GearActualPosn_enum/1 -> [VTQD_GearActualPosn_enum]
  [VTQD_TqTargetShaftSpd_rpm] -> ShiftD/3(VTQD_TqTargetShaftSpd_rpm)
  Equal7/1 -> GearShiftCheck/1
  GearShiftCheck/3 -> ShiftPorN/Action
  Equal8/1 -> GearShiftCheck/2
  [VTQD_ActAPSPosn_pct] -> ShiftR/1(VTQD_ActAPSPosn_pct)
  ShiftPorN/1(VTQD_PedalMapWhlTqPorN_Nm) -> Merge1/3
  [VTQD_EVDriveMode_enum] -> ShiftD/1(VTQD_EVDriveMode_enum)
  [VTQD_TqTargetShaftSpd_rpm] -> ShiftR/2(VTQD_TqTargetShaftSpd_rpm)
  GearShiftCheck/1 -> ShiftD/Action
  Merge1/1 -> VTQD_PedalMapWhlTqNoLHM_Nm/1  "VTQD_PedalMapWhlTqNoLHM_Nm"
  Constant12/1 -> Equal8/2
  Constant11/1 -> Equal7/2
  GearShiftCheck/2 -> ShiftR/Action
  [VTQD_GearActualPosn_enum] -> Equal7/1
  [VTQD_ActAPSPosn_pct] -> ShiftD/2(VTQD_ActAPSPosn_pct)
  [VTQD_GearActualPosn_enum] -> Equal8/1
  ShiftD/1(VTQD_PedalMapWhlTqD_Nm) -> Merge1/1
  VTQD_RollingShaftSpd_rpm/1 -> [VTQD_RollingShaftSpd_rpm]
  VTQD_RollRegenEnable_flg/1 -> [VTQD_RollRegenEnable_flg]
  VTQD_RegenMode_enum/1 -> [VTQD_RegenMode_enum]
  VTQD_ActAPSPosn_pct/1 -> [VTQD_ActAPSPosn_pct]
  VTQD_TqTargetShaftSpd_rpm/1 -> [VTQD_TqTargetShaftSpd_rpm]
  [VVMC_EstSlope_Deg] -> ShiftD/7(VVMC_EstSlope_Deg)
  [VTQD_APSReqTimer_s] -> ShiftD/8(VTQD_APSReqTimer_s)
  VVMC_EstSlope_Deg/1 -> [VVMC_EstSlope_Deg]
  VTQD_APSReqTimer_s/1 -> [VTQD_APSReqTimer_s]
  [VTQD_RegenMode_enum] -> ShiftD/4(VTQD_RegenMode_enum)
  [VTQD_LowIdleAccPedal_flg] -> ShiftD/9(VTQD_LowIdleAccPedal_flg)
  VTQD_LowIdleAccPedal_flg/1 -> [VTQD_LowIdleAccPedal_flg]
  VTQD_OPDHoldEnRel_flg/1 -> [VTQD_OPDHoldEnRel_flg]
  [VTQD_OPDHoldEnRel_flg] -> ShiftD/10(VTQD_OPDHoldEnRel_flg)
  VTQD_OPDHoldActRelTq_Nm/1 -> [VTQD_OPDHoldActRelTq_Nm]
  VTQD_VehActSpd_kph/1 -> [VTQD_VehActSpd_kph]
  [VTQD_OPDHoldActRelTq_Nm] -> ShiftD/11(VTQD_OPDHoldActRelTq_Nm)
  [VTQD_VehActSpd_kph] -> ShiftD/12(VTQD_VehActSpd_kph)
  VTQD_SlopeUp_flg/1 -> [VTQD_SlopeUp_flg]
  [VTQD_SlopeUp_flg] -> ShiftD/13(VTQD_SlopeUp_flg)
  VTQD_IVIRockModeEn_flg/1 -> [VTQD_IVIRockModeEn_flg]
  VINP_IVISnowModeCmd_flg/1 -> [VINP_IVISnowModeCmd_flg]
  [VINP_IVISnowModeCmd_flg] -> ShiftD/14(VINP_IVISnowModeCmd_flg)
  [VTQD_IVIRockModeEn_flg] -> ShiftD/15(VTQD_IVIRockModeEn_flg)
  [VTQD_PreDecTqLowLim_Nm] -> ShiftD/16(VTQD_PreDecTqLowLim_Nm)
  VTQD_PreDecTqLowLim_Nm/1 -> [VTQD_PreDecTqLowLim_Nm]
  VTQD_CreepEnable_flg/1 -> [VTQD_CreepEnable_flg]
  VTQD_BrkSwSta_flg/1 -> [VTQD_BrkSwSta_flg]
  [VTQD_CreepEnable_flg] -> ShiftD/18(VTQD_CreepEnable_flg)
  [VTQD_BrkSwSta_flg] -> ShiftD/17(VTQD_BrkSwSta_flg)

== system tqd/TQD/TorqueDemand/TorqueModule/DriverWhlTqDem/PedalMapWhlTq/Pedal G-Control Mode ==
  VINP_SCPSystemMode_enum : Inport
  VPMM_PwrSta_enum : Inport  Port=2
  VTQD_GearActualPosn_enum : Inport  Port=3
  VTQD_RegenMode_enum : Inport  Port=4
  VINP_SWC2RCustomizeSta_flg : Inport  Port=5
  task_time_s : Inport  Port=6
  VTQD_ActAPSPosn_pct : Inport  Port=7
  VTQD_TqTargetShaftSpd_rpm : Inport  Port=8
  VVMC_LongAcc_Gps : Inport  Port=9
  VINP_VehSpeed_kph : Inport  Port=10
  VTQD_CreepPrLoadEnable_flg : Inport  Port=11
  VINP_BrkPedalPos_pct : Inport  Port=12
  VINP_IVIPedalGRegenLim_pct : Inport  Port=13
  VVMC_SmartRegenReq_mps2 : Inport  Port=14
  VINP_IVISmartRegenSW_flg : Inport  Port=15
  VINP_IVICreepOnSW_flg : Inport  Port=16
  VTQD_APSReqTimer_s : Inport  Port=17
  VINP_SWCResUpSta_flg : Inport  Port=18
  Active Determination : Subsystem
  Torque Calculation : Subsystem
  VTQD_PedAccTqEn_flg : Outport
  VTQD_PedalTqCal_Nm : Outport  Port=2
  wires:
  Torque Calculation/1(VTQD_PedalTqCal_Nm) -> [VTQD_PedalTqCal_Nm]
  [VINP_VehSpeed_kph] -> Torque Calculation/4(VINP_VehSpeed_kph)
  [VTQD_ActAPSPosn_pct] -> Torque Calculation/1(VTQD_ActAPSPosn_pct)
  [VTQD_TqTargetShaftSpd_rpm] -> Torque Calculation/2(VTQD_TqTargetShaftSpd_rpm)
  [VTQD_PedAccTqEn_flg] -> Torque Calculation/5(VTQD_PedAccTqEn_flg)
  [VVMC_LongAcc_Gps] -> Torque Calculation/3(VVMC_LongAcc_Gps)
  Active Determination/1(VTQD_PedAccTqEn_flg) -> [VTQD_PedAccTqEn_flg]
  [VINP_SCPSystemMode_enum] -> Active Determination/1(VINP_SCPSystemMode_enum)
  [VPMM_PwrSta_enum] -> Active Determination/2(VPMM_PwrSta_enum)
  [VTQD_GearActualPosn_enum] -> Active Determination/3(VTQD_GearActualPosn_enum)
  [VTQD_RegenMode_enum] -> Active Determination/4(VTQD_RegenMode_enum)
  [VINP_SWC2RCustomizeSta_flg] -> Active Determination/5(VINP_SWC2RCustomizeSta_flg)
  [task_time_s] -> Active Determination/6(task_time_s)
  VTQD_GearActualPosn_enum/1 -> [VTQD_GearActualPosn_enum]
  VINP_SWC2RCustomizeSta_flg/1 -> [VINP_SWC2RCustomizeSta_flg]
  VPMM_PwrSta_enum/1 -> [VPMM_PwrSta_enum]
  task_time_s/1 -> [task_time_s]
  VINP_SCPSystemMode_enum/1 -> [VINP_SCPSystemMode_enum]
  VTQD_RegenMode_enum/1 -> [VTQD_RegenMode_enum]
  VTQD_ActAPSPosn_pct/1 -> [VTQD_ActAPSPosn_pct]
  VINP_VehSpeed_kph/1 -> [VINP_VehSpeed_kph]
  VVMC_LongAcc_Gps/1 -> [VVMC_LongAcc_Gps]
  VTQD_TqTargetShaftSpd_rpm/1 -> [VTQD_TqTargetShaftSpd_rpm]
  [VTQD_PedAccTqEn_flg] -> VTQD_PedAccTqEn_flg/1
  [VTQD_PedalTqCal_Nm] -> VTQD_PedalTqCal_Nm/1
  [VTQD_GearActualPosn_enum] -> Torque Calculation/6(VTQD_GearActualPosn_enum)
  VTQD_CreepPrLoadEnable_flg/1 -> [VTQD_CreepPrLoadEnable_flg]
  [VTQD_CreepPrLoadEnable_flg] -> Torque Calculation/7(VTQD_CreepPrLoadEnable_flg)
  [VINP_BrkPedalPos_pct] -> Torque Calculation/8(VINP_BrkPedalPos_pct)
  VINP_BrkPedalPos_pct/1 -> [VINP_BrkPedalPos_pct]
  [VINP_IVIPedalGRegenLim_pct] -> Torque Calculation/9(VINP_IVIPedalGRegenLim_pct)
  VINP_IVIPedalGRegenLim_pct/1 -> [VINP_IVIPedalGRegenLim_pct]
  [VVMC_SmartRegenReq_mps2] -> Torque Calculation/10(VVMC_SmartRegenReq_mps2)
  [VINP_IVISmartRegenSW_flg] -> Torque Calculation/11(VINP_IVISmartRegenSW_flg)
  VINP_IVISmartRegenSW_flg/1 -> [VINP_IVISmartRegenSW_flg]
  VVMC_SmartRegenReq_mps2/1 -> [VVMC_SmartRegenReq_mps2]
  [VINP_IVICreepOnSW_flg] -> Torque Calculation/12(VINP_IVICreepOnSW_flg)
  VINP_IVICreepOnSW_flg/1 -> [VINP_IVICreepOnSW_flg]
  [VTQD_APSReqTimer_s] -> Torque Calculation/13(VTQD_APSReqTimer_s)
  VTQD_APSReqTimer_s/1 -> [VTQD_APSReqTimer_s]
  VINP_SWCResUpSta_flg/1 -> [VINP_SWCResUpSta_flg]
  [VINP_SWCResUpSta_flg] -> Active Determination/7(VINP_SWCResUpSta_flg)

== system tqd/TQD/TorqueDemand/TorqueModule/DriverWhlTqDem/PedalMapWhlTq/Triggered Subsystem ==
  in1 : Inport
  In2 : Inport  Port=2
  Trigger : TriggerPort  VariantControl=(inherit)
  Out1 : Outport
  Out2 : Outport  Port=2
  wires:
  in1/1 -> Out1/1
  In2/1 -> Out2/1

== system tqd/TQD/TorqueDemand/Signal_convert/SWC2_Subsystem/Big Mike Combo/Combo Key Detection/DiagnosisOff Mode ==
  note: Exhibition Mode:
      | 1 = VINP_SWC2RegenDown_flg
      | 2 = VINP_SWC2RegenUp_flg
      | 3 = VINP_SWC2LScrollUpSta_flg
      | 4 = VINP_SWC2LScrollDownSta_flg
      | 5 = VINP_SWC2RScrollUpSta_flg
      | 6 = VINP_SWC2RScrollDownSta_flg
      | 7 = VINP_SWC2LScrollPressSta_flg
      | 8 = VINP_SWC2LADASSta_flg
  TASK_TIME_10_MS : Inport
  VSCP_ComboKeyEn_flg : Inport  Port=2
  VSCP_ComboKeyReset_flg : Inport  Port=3
  VSCP_ComboKey_enum : Inport  Port=4
  VSCP_ComboKeyEnter_flg : Inport  Port=5
  VSCP_StreetFightModeOff_flg : Inport  Port=6
  AND : Logic  Inputs=9  AllPortsSameDT=off  OutDataTypeStr=boolean
  Constant : Constant  Value=ENUM_COMBOKEY_NONE
  Constant1 : Constant  Value=ENUM_COMBOKEY_NONE
  Constant2 : Constant  Value=FALSE
  Constant3 : Constant  Value=KTQD_ComboKeyDelay_s
  Delay : Delay  DelayLength=1
  DelayEnable : hcu_lib/Basic_Blocks/DelayEnable
  Equal : RelationalOperator  Operator=~=  OutDataTypeStr=boolean  RndMeth=Simplest
  Key1 : Subsystem
  Key2 : Subsystem
  Key3 : Subsystem
  Key4 : Subsystem
  Key5 : Subsystem
  Key6 : Subsystem
  Key7 : Subsystem
  Key8 : Subsystem
  Switch : Switch  Criteria=u2 > Threshold
  Switch1 : Switch  Criteria=u2 > Threshold
  Switch2 : Switch  Criteria=u2 > Threshold
  VSCP_DiagnosisOffMode_flg : Outport
  wires:
  [VSCP_ComboKey8_enum] -> Equal/1
  Key7/1(VSCP_ComboKey7_enum) -> [VSCP_ComboKey7_enum]
  Key6/2(VSCP_Key6Pass_flg) -> [VSCP_Key6Pass_flg]
  Key6/1(VSCP_ComboKey6_enum) -> [VSCP_ComboKey6_enum]
  VSCP_StreetFightModeOff_flg/1 -> [VSCP_StreetFightModeOff_flg]
  VSCP_ComboKeyEnter_flg/1 -> [VSCP_ComboKeyEnter_flg]
  VSCP_ComboKey_enum/1 -> [VSCP_ComboKey_enum]
  VSCP_ComboKeyReset_flg/1 -> [VSCP_ComboKeyReset_flg]
  VSCP_ComboKeyEn_flg/1 -> [VSCP_ComboKeyEn_flg]
  TASK_TIME_10_MS/1 -> [TASK_TIME_10_MS]
  Delay/1 -> Switch1/3
  Switch2/1 -> [VSCP_DiagnosisOffMode_flg], Delay/1  "VTQD_DiagnosisOffMode_flg"
  Constant2/1 -> Switch2/1
  [VSCP_StreetFightModeOff_flg] -> Switch2/2
  Switch1/1 -> Switch2/3
  AND/1 -> Switch1/1  "VTQD_DiagnosisOffPass_flg"
  [VSCP_ComboKeyEnter_flg] -> Switch1/2
  [VSCP_Key2Pass_flg] -> AND/3
  [VSCP_Key3Pass_flg] -> AND/4
  [VSCP_Key4Pass_flg] -> AND/5
  [VSCP_Key5Pass_flg] -> AND/6
  [VSCP_Key6Pass_flg] -> AND/7
  [VSCP_Key7Pass_flg] -> AND/8
  [VSCP_Key8Pass_flg] -> AND/9
  [VSCP_Key1Pass_flg] -> AND/2
  Equal/1 -> AND/1
  Constant1/1 -> Equal/2
  [VSCP_ComboKey7_enum] -> Key8/4(VSCP_ComboKey7_enum)
  [VSCP_ComboKeyReset_flg] -> Key8/3(VSCP_ComboKeyReset_flg)
  [VSCP_ComboKeyEn_flg] -> Key8/2(VSCP_ComboKeyEn_flg)
  [VSCP_ComboKeyCMD_enum] -> Key8/1(VSCP_ComboKeyCMD_enum)
  [VSCP_ComboKey6_enum] -> Key7/4(VSCP_ComboKey6_enum)
  [VSCP_ComboKeyReset_flg] -> Key7/3(VSCP_ComboKeyReset_flg)
  [VSCP_ComboKeyEn_flg] -> Key7/2(VSCP_ComboKeyEn_flg)
  [VSCP_ComboKeyCMD_enum] -> Key7/1(VSCP_ComboKeyCMD_enum)
  [VSCP_ComboKey5_enum] -> Key6/4(VSCP_ComboKey5_enum)
  [VSCP_ComboKeyReset_flg] -> Key6/3(VSCP_ComboKeyReset_flg)
  [VSCP_ComboKeyEn_flg] -> Key6/2(VSCP_ComboKeyEn_flg)
  [VSCP_ComboKeyCMD_enum] -> Key6/1(VSCP_ComboKeyCMD_enum)
  Key8/2(VSCP_Key8Pass_flg) -> [VSCP_Key8Pass_flg]
  Key8/1(VSCP_ComboKey8_enum) -> [VSCP_ComboKey8_enum]
  Key7/2(VSCP_Key7Pass_flg) -> [VSCP_Key7Pass_flg]
  Key5/1(VSCP_ComboKey5_enum) -> [VSCP_ComboKey5_enum]
  Key5/2(VSCP_Key5Pass_flg) -> [VSCP_Key5Pass_flg]
  [VSCP_ComboKey4_enum] -> Key5/4(VSCP_ComboKey4_enum)
  [VSCP_ComboKeyCMD_enum] -> Key5/1(VSCP_ComboKeyCMD_enum)
  [VSCP_ComboKeyEn_flg] -> Key5/2(VSCP_ComboKeyEn_flg)
  [VSCP_ComboKeyReset_flg] -> Key5/3(VSCP_ComboKeyReset_flg)
  Key4/2(VSCP_Key4Pass_flg) -> [VSCP_Key4Pass_flg]
  Key4/1(VSCP_ComboKey4_enum) -> [VSCP_ComboKey4_enum]
  Key3/2(VSCP_Key3Pass_flg) -> [VSCP_Key3Pass_flg]
  Key3/1(VSCP_ComboKey3_enum) -> [VSCP_ComboKey3_enum]
  [VSCP_ComboKey3_enum] -> Key4/4(VSCP_ComboKey3_enum)
  Key2/2(VSCP_Key2Pass_flg) -> [VSCP_Key2Pass_flg]
  Key2/1(VSCP_ComboKey2_enum) -> [VSCP_ComboKey2_enum]
  [VSCP_ComboKeyReset_flg] -> Key4/3(VSCP_ComboKeyReset_flg)
  [VSCP_ComboKeyEn_flg] -> Key4/2(VSCP_ComboKeyEn_flg)
  [VSCP_ComboKeyCMD_enum] -> Key4/1(VSCP_ComboKeyCMD_enum)
  [VSCP_ComboKey2_enum] -> Key3/4(VSCP_ComboKey2_enum)
  [VSCP_ComboKeyReset_flg] -> Key3/3(VSCP_ComboKeyReset_flg)
  [VSCP_ComboKeyEn_flg] -> Key3/2(VSCP_ComboKeyEn_flg)
  [VSCP_ComboKeyCMD_enum] -> Key3/1(VSCP_ComboKeyCMD_enum)
  Key1/2(VSCP_Key1Pass_flg) -> [VSCP_Key1Pass_flg]
  Key1/1(VSCP_ComboKey1_enum) -> [VSCP_ComboKey1_enum]
  [VSCP_ComboKey1_enum] -> Key2/4(VSCP_ComboKey1_enum)
  [VSCP_ComboKeyReset_flg] -> Key2/3(VSCP_ComboKeyReset_flg)
  [VSCP_ComboKeyEn_flg] -> Key2/2(VSCP_ComboKeyEn_flg)
  [VSCP_ComboKeyCMD_enum] -> Key2/1(VSCP_ComboKeyCMD_enum)
  [VSCP_ComboKeyReset_flg] -> Key1/3(VSCP_ComboKeyReset_flg)
  [VSCP_ComboKeyEn_flg] -> Key1/2(VSCP_ComboKeyEn_flg)
  [VSCP_ComboKeyCMD_enum] -> Key1/1(VSCP_ComboKeyCMD_enum)
  [VSCP_ComboKey_enum] -> Switch/1
  Constant3/1 -> DelayEnable/2
  [VSCP_ComboKeyEn_flg] -> DelayEnable/1
  DelayEnable/1 -> Switch/2
  Constant/1 -> Switch/3
  [TASK_TIME_10_MS] -> DelayEnable/3
  Switch/1 -> [VSCP_ComboKeyCMD_enum]  "VTQD_DiagnosisOffCMD_enum"
  [VSCP_DiagnosisOffMode_flg] -> VSCP_DiagnosisOffMode_flg/1
